simulink model "questao6_simulink"  (Simulink 9.1)
settings: Solver=VariableStepAuto  StartTime=0.0  StopTime=10.0  RelTol=1e-3
settings Model: Creator=wLeon  LastModifiedBy=wLeon
settings DataIOCC: SaveFormat=Dataset
settings OptimizationCC: LifeSpan=auto
settings DebuggingCC: UnderspecifiedInitializationDetection=Simplified  MergeDetectMultiDrivingBlocksExec=error  SFUnexpectedBacktrackingDiag=error  SFNoUnconditionalDefaultTransitionDiag=error  SFExecutionAtInitializationDiag=warning
settings HardwareCC: ProdBitPerPointer=64  ProdBitPerSizeT=64  ProdBitPerPtrDiffT=64  ProdLargestAtomicFloat=Float  ProdIntDivRoundTo=Zero  ProdEndianess=LittleEndian  ProdWordSize=64  ProdHWDeviceType=Intel->x86-64 (Windows64)
settings ModelReferenceCC: PropagateSignalLabelsOutOfModel=on
settings CodeAppCC: StateflowObjectComments=off
settings GRTTargetCC: TargetLangStandard=C99 (ISO)  CombineOutputUpdateFcns=on  GRTInterface=off
settings ConfigComp: CovMetricSettings=dwe  CovHtmlReporting=off  CovSaveCumulativeToWorkspaceVar=off  CovSaveSingleToWorkspaceVar=off  CovExternalEMLEnable=on

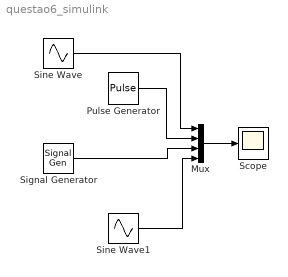
== system questao6_simulink ==
  Mux : Mux
  Pulse Generator : DiscretePulseGenerator  PulseType=Time based  Amplitude=3  Period=1  PulseWidth=5
      settings: AttributesFormatString=|
      | Amplitude: %<Amplitude>
      | Periodo: %<Period>
  Scope : Scope
      settings: AttributesFormatString=%<Description>
  Signal Generator : SignalGenerator  WaveForm=square  Amplitude=8  Frequency=10  Units=rad/sec
      settings: AttributesFormatString=|
      | Amplitude: %<Amplitude>
      | Frequencia: %<Frequency>
  Sine Wave : Sin  Amplitude=5  SampleTime=0
      settings: AttributesFormatString=|
      | Amplitude: %<Amplitude>
      | Frequencia: %<Frequency>
  Sine Wave1 : Sin  SampleTime=0
      settings: AttributesFormatString=|
      | Amplitude: %<Amplitude>
      | Frequencia: %<Frequency>
  wires:
  Sine Wave/1 -> Mux/1
  Pulse Generator/1 -> Mux/2
  Signal Generator/1 -> Mux/3
  Sine Wave1/1 -> Mux/4
  Mux/1 -> Scope/1
